simulink model "tarea1_jevg"  (R2021a)
settings: Solver=VariableStepAuto  StartTime=0.0  StopTime=10  RelTol=1e-3
libraries: fl_lib x8, nesl_utility x3
settings Model: LastModifiedBy=user
settings DebuggingCC: UnconnectedInputMsg=none  UnconnectedOutputMsg=none  UnconnectedLineMsg=none
settings ModelReferenceCC: EnableRefExpFcnMdlSchedulingChecks=off
settings RTWCC: Description=Generic Real-Time Target  DLArmComputeVersion=20.02.1

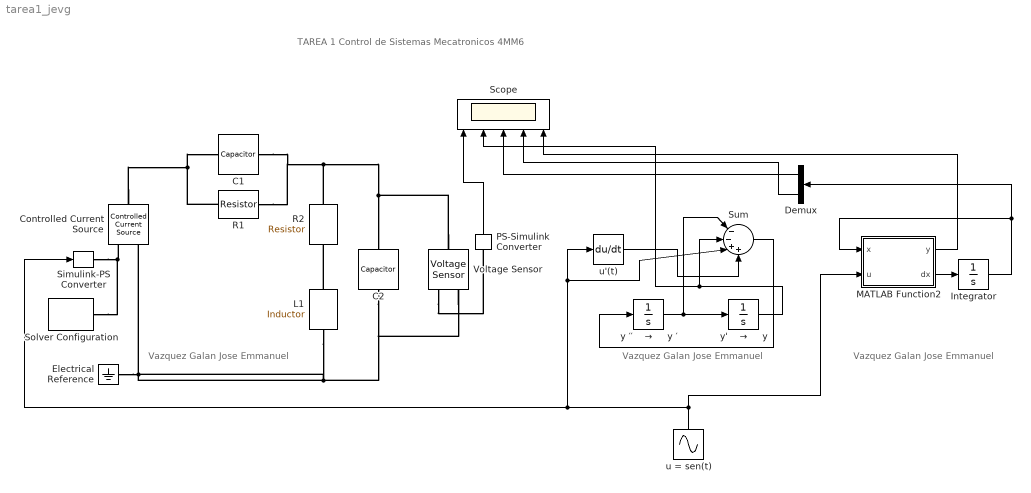
== system tarea1_jevg ==
  note: TAREA 1
      | Control de Sistemas Mecatronicos 4MM6
  note: Vazquez Galan Jose Emmanuel
  note: Vazquez Galan Jose Emmanuel
  note: Vazquez Galan Jose Emmanuel
  C1 : fl_lib/Electrical/Electrical Elements/Capacitor  c=1 F  r=1e-6 Ohm  g=0 1/Ohm  i_specify=off  i_priority=None  i=0 A  i_nominal_specify=off  i_nominal_unit=A  i_nominal_value=1  v_specify=off  v_priority=None  v=0 V  v_nominal_specify=off  v_nominal_unit=V  v_nominal_value=1  vc_specify=off  vc_priority=High  vc=0 V  vc_nominal_specify=off  vc_nominal_unit=V  vc_nominal_value=1
  C2 : fl_lib/Electrical/Electrical Elements/Capacitor  c=1 F  r=1e-6 Ohm  g=0 1/Ohm  i_specify=off  i_priority=None  i=0 A  i_nominal_specify=off  i_nominal_unit=A  i_nominal_value=1  v_specify=off  v_priority=None  v=0 V  v_nominal_specify=off  v_nominal_unit=V  v_nominal_value=1  vc_specify=off  vc_priority=High  vc=0 V  vc_nominal_specify=off  vc_nominal_unit=V  vc_nominal_value=1
  Controlled Current Source : fl_lib/Electrical/Electrical Sources/Controlled Current Source
  Demux : Demux  Outputs=2
  Electrical Reference : fl_lib/Electrical/Electrical Elements/Electrical Reference
  Integrator : Integrator  InitialCondition=[0 0]'
  L1 : fl_lib/Electrical/Electrical Elements/Inductor  l=1 H  r=0 Ohm  g=1e-9 1/Ohm  i_specify=off  i_priority=None  i=0 A  i_nominal_specify=off  i_nominal_unit=A  i_nominal_value=1  v_specify=off  v_priority=None  v=0 V  v_nominal_specify=off  v_nominal_unit=V  v_nominal_value=1  i_L_specify=off  i_L_priority=High  i_L=0 A  i_L_nominal_specify=off  i_L_nominal_unit=A  i_L_nominal_value=1
  MATLAB Function2 : MATLAB Function  TreatAsAtomicUnit=on
  PS-Simulink Converter : nesl_utility/PS-Simulink Converter  PhysicalDomain=network_engine_domain  SubClassName=ps_output  LeftPortType=input  RightPortType=output  PseudoPeriodic=off  Frequencies=[]  Unit=inherit  AffineConversion=off
      settings: SourceProductBaseCode=PW,SS
  R1 : fl_lib/Electrical/Electrical Elements/Resistor  R=1 Ohm  i_specify=off  i_priority=None  i=0 A  i_nominal_specify=off  i_nominal_unit=A  i_nominal_value=1  v_specify=off  v_priority=None  v=0 V  v_nominal_specify=off  v_nominal_unit=V  v_nominal_value=1
  R2 : fl_lib/Electrical/Electrical Elements/Resistor  R=1 Ohm  i_specify=off  i_priority=None  i=0 A  i_nominal_specify=off  i_nominal_unit=A  i_nominal_value=1  v_specify=off  v_priority=None  v=0 V  v_nominal_specify=off  v_nominal_unit=V  v_nominal_value=1
  Scope : Scope  NumInputPorts=5
  Simulink-PS Converter : nesl_utility/Simulink-PS Converter  PhysicalDomain=network_engine_domain  SubClassName=ps_input  LeftPortType=input  RightPortType=output  PseudoPeriodic=off  Frequencies=[]  NoiseDistribution=none  NoiseParameters=[]  Unit=1  AffineConversion=off  FilteringAndDerivatives=provide  SimscapeFilterOrder=1  InputFilterTimeConstant=0.001  UdotUserProvided=0
      settings: SourceProductBaseCode=PW,SS
  Solver Configuration : nesl_utility/Solver Configuration  PhysicalDomain=network_engine_domain  SubClassName=solver  LeftPortType=input  RightPortType=generic  Tones=[]  Harmonics=[]  SimulateNoise=off  Profile=off  UseLocalSampling=off  EnableSwitchedLinearOptims=on  FrequencyDomain=off  UseCCode=off  RelTol=0.001  AbsTol=0.001  MinStep=1e-09  ToWorkspace=off  RevertToSquareIcSolve=off  NumHomotopyIterations=100  PhasorMode=off  PhasorModeNumHarmonics=1  DoDC=on  ResidualTolerance=1e-09  UseLocalSolver=off  LocalSolverChoice=NE_BACKWARD_EULER_ADVANCER  LocalSolverSampleTime=0.001  DoFixedCost=off  MaxNonlinIter=3  MaxModeIter=2  ComputeImpulses=off  ImpulseIterations=2  LinearAlgebra=auto  EquationFormulation=NE_TIME_EF  DelaysMemoryBudget=1024  AutomaticFiltering=on  FilteringTimeConstant=0.001  PartitionStorageMethod=AS_NEEDED  PartitionMemoryBudget=1024  PartitionMethod=ROBUST
      settings: SourceProductBaseCode=PW,SS
  Sum : Sum  Inputs=|--++
  Voltage Sensor : fl_lib/Electrical/Electrical Sensors/Voltage Sensor
  "u = sen(t) " : Sin  SampleTime=0
  u'(t) : Derivative
  y ′′    →     y ′ : Integrator
  y'    →     y : Integrator
  wires:
  PS-Simulink Converter/1 -> Scope/1
  "u = sen(t) "/1 -> MATLAB Function2/2(u), Sum/3, u'(t)/1, Simulink-PS Converter/1
  y ′′    →     y ′/1 -> y'    →     y/1, Sum/1
  y'    →     y/1 -> Sum/2, Scope/2
  Sum/1 -> y ′′    →     y ′/1
  MATLAB Function2/2(dx) -> Integrator/1
  Integrator/1 -> Demux/1, MATLAB Function2/1(x)
  MATLAB Function2/1(y) -> Scope/5
  Demux/1 -> Scope/3
  Demux/2 -> Scope/4
  u'(t)/1 -> Sum/4
  connections:
  R2/LConn1 -- R1/RConn1 -- C1/RConn1 -- Voltage Sensor/LConn1 -- C2/LConn1
  L1/LConn1 -- R2/RConn1
  R1/LConn1 -- Controlled Current Source/LConn1 -- C1/LConn1
  Electrical Reference/LConn1 -- L1/RConn1 -- Voltage Sensor/RConn2 -- C2/RConn1 -- Controlled Current Source/RConn2
  Voltage Sensor/RConn1 -- PS-Simulink Converter/LConn1
  Simulink-PS Converter/RConn1 -- Solver Configuration/RConn1 -- Controlled Current Source/RConn1

== matlab function tarea1_jevg/MATLAB Function2 ==
  data: x input; u input; y output; dx output
function [y,dx] = fcn(x,u)

    A = [0 1; -1 -1];
    B = [1; 0];
    C=  [1 0];

dx = A*x+B*u;
y = C*x;
